simulink model "PFC"  (R2018b)
settings: Solver=VariableStepAuto  StartTime=0.0  StopTime=8  MaxStep=1e-4  RelTol=1e-3
values from neighbouring files (symbols this model uses):
  C = 470e-6    (= 0.00047)    [Parameter_DAD.m]    (also in Parameter_PFC.m = 7.2e-10)
  f_ac = 50    [Parameter_PFC.m]
  I_u = 10    [Parameter_DAD.m]    (also in Parameter_PFC.m)
  L = 50*1e-4    (= 0.005)    [Parameter_DAD.m]    (also in Parameter_PFC.m = 0.003)
  P_u = 5    [Parameter_DAD.m]    (also in Parameter_PFC.m = 0.1)
  R_l = Vdc_trgt^2 / P/eita    (= 400)    [Parameter_PFC.m]
  Vac = 220    [Parameter_PFC.m]
  Vdc_trgt = 400    [Parameter_PFC.m]
libraries: powerlib x16, simulink_extras x2, simulink x1
settings Model: Creator=lenovo  LastModifiedBy=lenovo
settings SFSimCC: SimUseLocalCustomCode=off
settings RTWCC: RTWUseLocalCustomCode=off
settings CodeAppCC: StateflowObjectComments=on

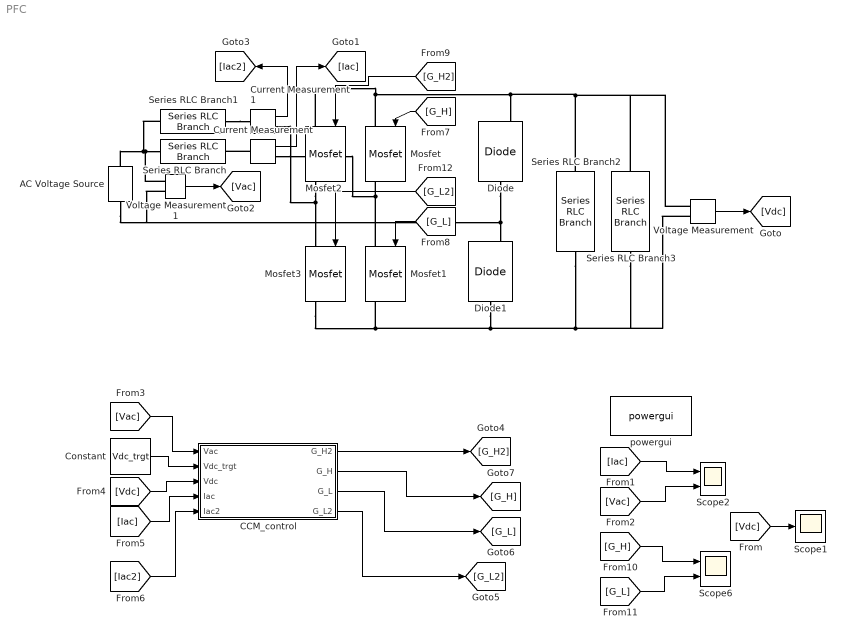
== system PFC ==
  AC Voltage Source : powerlib/Electrical Sources/AC Voltage Source  Amplitude=Vac*sqrt(2)  Phase=0  Frequency=f_ac  SampleTime=0  Measurements=None  BusType=swing  Pref=10e3  Qref=0  Qmin=-inf  Qmax=+inf
      settings: SourceProductName=Simscape Electrical
  CCM_control : Subsystem
  Constant : Constant  Value=Vdc_trgt
  Current Measurement : powerlib/Measurements/Current Measurement  PhasorSimulation=off  OutputType=Complex  PSBequivalent=0
  Current Measurement1 : powerlib/Measurements/Current Measurement  PhasorSimulation=off  OutputType=Complex  PSBequivalent=0
  Diode : powerlib/Power Electronics/Diode  Ron=0.001  Lon=0  Vf=0.8  IC=0  UseSnubber=0  Rs=500  Cs=250e-9  Measurements=on
      settings: SourceProductName=Simscape Electrical
  Diode1 : powerlib/Power Electronics/Diode  Ron=0.001  Lon=0  Vf=0.8  IC=0  UseSnubber=0  Rs=500  Cs=250e-9  Measurements=on
      settings: SourceProductName=Simscape Electrical
  Mosfet{,1..3} (4 alike) : powerlib/Power Electronics/Mosfet  Ron=0.1  Lon=0  Rd=0.01  Vfd=0  IC=0  Rs=1e5  Cs=inf  Measurements=on
      settings: SourceProductName=Simscape Electrical
  Scope1 : Scope
  Scope2 : Scope  NumInputPorts=2
  Scope6 : Scope  NumInputPorts=2
  Series RLC Branch : powerlib/Elements/Series RLC Branch  LConnTagsString=__new0  RConnTagsString=__new0  BranchType=L  Resistance=1  Inductance=L  SetiL0=off  InitialCurrent=0  Capacitance=1e-6  Setx0=off  InitialVoltage=0  Measurements=None
      settings: SourceProductName=Simscape Electrical
  Series RLC Branch1 : powerlib/Elements/Series RLC Branch  LConnTagsString=__new0  RConnTagsString=__new0  BranchType=L  Resistance=1  Inductance=L  SetiL0=off  InitialCurrent=0  Capacitance=1e-6  Setx0=off  InitialVoltage=0  Measurements=None
      settings: SourceProductName=Simscape Electrical
  Series RLC Branch2 : powerlib/Elements/Series RLC Branch  LConnTagsString=__new0  RConnTagsString=__new0  BranchType=C  Resistance=1  Inductance=1e-3  SetiL0=off  InitialCurrent=0  Capacitance=C  Setx0=on  InitialVoltage=0  Measurements=None
      settings: SourceProductName=Simscape Electrical
  Series RLC Branch3 : powerlib/Elements/Series RLC Branch  LConnTagsString=__new0  RConnTagsString=__new0  BranchType=R  Resistance=R_l  Inductance=1e-3  SetiL0=off  InitialCurrent=0  Capacitance=C  Setx0=off  InitialVoltage=0  Measurements=None
      settings: SourceProductName=Simscape Electrical
  Voltage Measurement : powerlib/Measurements/Voltage Measurement  PhasorSimulation=off  OutputType=Complex  PSBequivalent=0
  Voltage Measurement1 : powerlib/Measurements/Voltage Measurement  PhasorSimulation=off  OutputType=Complex  PSBequivalent=0
  powergui : powerlib/powergui  Priority=1  SimulationMode=Discrete  SampleTime=1e-7  frequency=60  Iterations=50  frequencyindice=50  Pbase=100e6  ErrMax=1e-4  UnitsV=kV  UnitsW=MW  buscounter=0  FunctionMessages=off  echomessages=off  EnableUseOfTLC=off  CurrentSourceSwitches=off  DisableSnubberDevices=off  DisableRonSwitches=off  DisableVfSwitches=off  DisplayEquations=off  SolverType=Tustin/Backward Euler (TBE)  Interpol=off  ExternalGateDelay=off  methode=off  Ts=100  x0status=blocks  SPID=off  SwTol=0  HookPort=off  RestoreLinks=warning  ResistiveCurrentMeasurement=off  Frange=[0:2:500]  Ylog=off  Xlog=on  ShowGrid=off  save=off  variable=ZData  structure=0  ZoomFFT=off  StartTime=0.0  cycles=1  DisplayStyle=1  fundamental=60  FreqAxis=off  MaxFrequency=1000  frequencyindicesteady=1  RmsSteady=1  display=off
  wires:
  Voltage Measurement/1 -> [Vdc]
  [Vdc] -> Scope1/1
  Current Measurement/1 -> [Iac]
  [Iac] -> Scope2/1
  Voltage Measurement1/1 -> [Vac]
  [Vac] -> Scope2/2
  [G_H] -> Mosfet/1
  [G_L] -> Mosfet1/1
  [G_H] -> Scope6/1
  [G_L] -> Scope6/2
  [Vac] -> CCM_control/1(Vac)
  Constant/1 -> CCM_control/2(Vdc_trgt)
  [Vdc] -> CCM_control/3(Vdc)
  [Iac] -> CCM_control/4(Iac)
  CCM_control/2(G_H) -> [G_H]
  CCM_control/3(G_L) -> [G_L]
  Current Measurement1/1 -> [Iac2]
  [G_H2] -> Mosfet2/1
  [G_L2] -> Mosfet3/1
  [Iac2] -> CCM_control/5(Iac2)
  CCM_control/1(G_H2) -> [G_H2]
  CCM_control/4(G_L2) -> [G_L2]
  connections:
  Mosfet1/LConn1 -- Current Measurement/RConn1 -- Mosfet/RConn1
  Diode/LConn1 -- Voltage Measurement1/LConn2 -- AC Voltage Source/LConn1 -- Diode1/RConn1
  Diode1/LConn1 -- Voltage Measurement/LConn2 -- Series RLC Branch3/RConn1 -- Series RLC Branch2/RConn1 -- Mosfet3/RConn1 -- Mosfet1/RConn1
  Mosfet/LConn1 -- Mosfet2/LConn1 -- Voltage Measurement/LConn1 -- Series RLC Branch3/LConn1 -- Series RLC Branch2/LConn1 -- Diode/RConn1
  AC Voltage Source/RConn1 -- Series RLC Branch1/LConn1 -- Series RLC Branch/LConn1 -- Voltage Measurement1/LConn1
  Current Measurement/LConn1 -- Series RLC Branch/RConn1
  Series RLC Branch1/RConn1 -- Current Measurement1/LConn1
  Mosfet2/RConn1 -- Mosfet3/LConn1 -- Current Measurement1/RConn1

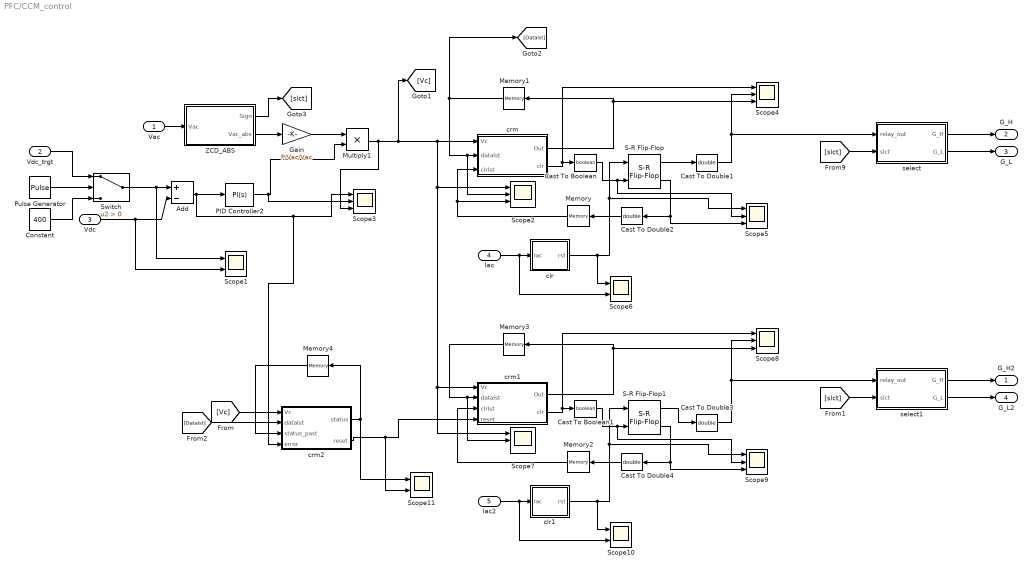
== system PFC/CCM_control ==
  Vac : Inport
  Vdc_trgt : Inport  Port=2
  Vdc : Inport  Port=3
  Iac : Inport  Port=4
  Iac2 : Inport  Port=5
  Add : Sum  Inputs=+-
  Cast To Boolean : DataTypeConversion  OutDataTypeStr=boolean
  Cast To Boolean1 : DataTypeConversion  OutDataTypeStr=boolean
  Cast To Double{1..4} (4 alike) : DataTypeConversion  OutDataTypeStr=double
  Constant : Constant  Value=400
  Gain : Gain  Gain=P/Vac/Vac
  Memory{,1..4} (5 alike) : Memory
  Multiply1 : Product
  PID Controller2 : simulink/Continuous/PID Controller  Controller=PI  Form=Parallel  TimeDomain=Continuous-time  SampleTime=-1  IntegratorMethod=Forward Euler  FilterMethod=Forward Euler  ControllerParametersSource=internal  P=P_u  I=I_u  D=0  UseFilter=on  N=100  TunerSelectOption=Transfer Function Based (PID Tuner App)  InitialConditionSource=internal  InitialConditionForIntegrator=0  InitialConditionForFilter=0  DifferentiatorICPrevScaledInput=0  ExternalReset=none  TrackingMode=off  Kt=1  LimitOutput=on  UpperSaturationLimit=50  LowerSaturationLimit=-10  LinearizeAsGain=off  AntiWindupMode=none  Kb=1  POutMin=[]  POutMax=[]  IOutMin=[]  IOutMax=[]  DOutMin=[]  DOutMax=[]  NOutMin=[]  NOutMax=[]  SumOutMin=[]  SumOutMax=[]  SaturationOutMin=[]  SaturationOutMax=[]  PParamMin=[]  PParamMax=[]  IParamMin=[]  IParamMax=[]  DParamMin=[]  DParamMax=[]  NParamMin=[]  NParamMax=[]  KbParamMin=[]  KbParamMax=[]  KtParamMin=[]  KtParamMax=[]  KbOutMin=[]  KbOutMax=[]  KtOutMin=[]  KtOutMax=[]  IntegratorOutMin=[]  IntegratorOutMax=[]  FilterOutMin=[]  FilterOutMax=[]  SumI1OutMin=[]  SumI1OutMax=[]  SumI2OutMin=[]  SumI2OutMax=[]  SumI3OutMin=[]  SumI3OutMax=[]  SumI4OutMin=[]  SumI4OutMax=[]  SumDOutMin=[]  SumDOutMax=[]  DifferentiatorOutMin=[]  DifferentiatorOutMax=[]  FilterDiffOutCoefMin=[]  FilterDiffOutCoefMax=[]  ReciprocalOutMin=[]  ReciprocalOutMax=[]  SumDenOutMin=[]  SumDenOutMax=[]  SumNumOutMin=[]  SumNumOutMax=[]  DivideOutMin=[]  DivideOutMax=[]  IntegratorContinuousStateAttributes=''  IntegratorStateMustResolveToSignalObject=off  IntegratorRTWStateStorageClass=Auto  FilterContinuousStateAttributes=''  FilterStateMustResolveToSignalObject=off  FilterRTWStateStorageClass=Auto  ParallelPVariant=InternalParameters  IdealPVariant=Disabled  IVariant=InternalParameters  DVariant=Disabled  IntegratorVariant=Continuous  SatVariant=Enabled  AWVariant=Passthrough  PCopyVariant=Disabled  TRVariant=Disabled  FdbkBlocksVariant=Forward  IdealPFdbkVariant=Disabled  SatFdbkVariant=Disabled  DerivativeFilterVariant=Disabled  NVariant=Disabled  NCopyVariant=Disabled_SignalSpec  FilterICVariant=Disabled  IntegratorICVariant=InternalICs  ExternalResetVariant=Disabled  TRSumVariant=Passthrough  SumFdbkVariant=Disabled  SumVariant=Sum_PI
  Pulse Generator : DiscretePulseGenerator  PulseType=Time based  Period=4  PulseWidth=50
  S-R Flip-Flop : simulink_extras/Flip Flops/S-R Flip-Flop  initial_condition=0
  S-R Flip-Flop1 : simulink_extras/Flip Flops/S-R Flip-Flop  initial_condition=0
  Scope{1,6,10..11} (4 alike) : Scope  NumInputPorts=2
  Scope{2..5,7..9} (7 alike) : Scope  NumInputPorts=3
  Switch : Switch  Criteria=u2 > Threshold
  ZCD_ABS : MATLAB Function  TreatAsAtomicUnit=on
  clr : MATLAB Function  TreatAsAtomicUnit=on
  clr1 : MATLAB Function  TreatAsAtomicUnit=on
  crm : MATLAB Function  TreatAsAtomicUnit=on
  crm1 : MATLAB Function  TreatAsAtomicUnit=on
  crm2 : MATLAB Function  TreatAsAtomicUnit=on
  select : MATLAB Function  TreatAsAtomicUnit=on
  select1 : MATLAB Function  TreatAsAtomicUnit=on
  G_H2 : Outport
  G_H : Outport  Port=2
  G_L : Outport  Port=3
  G_L2 : Outport  Port=4
  wires:
  select/2(G_L) -> G_L/1
  ZCD_ABS/2(Vac_abs) -> Gain/1
  select/1(G_H) -> G_H/1
  Add/1 -> crm2/4(error), Scope3/1, PID Controller2/1
  PID Controller2/1 -> Scope3/2, Multiply1/2
  ZCD_ABS/1(Sign) -> [slct]
  Gain/1 -> Multiply1/1
  [slct] -> select/2(slct)
  Vac/1 -> ZCD_ABS/1(Vac)
  Vdc/1 -> Scope1/2, Add/2
  Pulse Generator/1 -> Switch/2
  Constant/1 -> Switch/3
  Vdc_trgt/1 -> Switch/1
  Switch/1 -> Scope1/1, Add/1
  crm/1(Out) -> Scope4/3, Memory1/1
  Memory/1 -> crm/3(clrlst), Scope2/3
  Cast To Double1/1 -> select/1(relay_out), Scope4/2
  Cast To Double2/1 -> Memory/1
  crm/2(clr) -> Scope4/1, Cast To Boolean/1
  Iac/1 -> Scope6/2, clr/1(Iac)
  S-R Flip-Flop/1 -> Cast To Double1/1
  S-R Flip-Flop/2 -> Scope5/3, Cast To Double2/1
  clr/1(rst) -> Scope6/1, Scope5/1, S-R Flip-Flop/1
  Cast To Boolean/1 -> Scope5/2, S-R Flip-Flop/2
  S-R Flip-Flop1/2 -> Scope9/3, Cast To Double4/1
  Cast To Boolean1/1 -> Scope9/2, S-R Flip-Flop1/2
  crm1/2(clr) -> Scope8/1, Cast To Boolean1/1
  clr1/1(rst) -> Scope10/1, Scope9/1, S-R Flip-Flop1/1
  Iac2/1 -> Scope10/2, clr1/1(Iac)
  [slct] -> select1/2(slct)
  select1/2(G_L) -> G_L2/1
  Multiply1/1 -> Scope3/3, [Vc], Scope7/1, crm1/1(Vc), Scope2/1, crm/1(Vc)
  Cast To Double4/1 -> Memory2/1
  select1/1(G_H) -> G_H2/1
  Cast To Double3/1 -> select1/1(relay_out), Scope8/2
  S-R Flip-Flop1/1 -> Cast To Double3/1
  Memory3/1 -> Scope7/2, crm1/2(datalst)
  crm1/1(Out) -> Scope8/3, Memory3/1
  Memory2/1 -> crm1/3(clrlst)
  Memory4/1 -> crm2/3(status_past)
  [Vc] -> crm2/1(Vc)
  Memory1/1 -> [Datalst], Scope2/2, crm/2(datalst)
  [Datalst] -> crm2/2(datalst)
  crm2/1(status) -> Memory4/1, Scope11/1
  crm2/2(reset) -> Scope11/2, crm1/4(reset)

== matlab function PFC/CCM_control/select ==
  data: relay_out input; G_H output; G_L output; slct input
function [G_H, G_L] = fcn(relay_out, slct)


if slct>0.5
    G_L = relay_out;
    G_H = 1-relay_out;
elseif slct<=-0.5
    G_L = 1-relay_out;
    G_H = relay_out; 
else
    G_L = 0;
    G_H = 0; 
end    
end

== matlab function PFC/CCM_control/ZCD_ABS ==
  data: Vac input; Sign output; Vac_abs output
function [Sign, Vac_abs] = fcn(Vac)
Vac_abs = abs(Vac);
Sign = sign(Vac);
end

== matlab function PFC/CCM_control/crm ==
  data: Vc input size=1; Out output size=1; datalst input size=1; clr output size=1; clrlst input size=1
function [Out, clr] = fcn(Vc, datalst, clrlst)
if Vc <= datalst
    clr = 1;
else
    clr = 0;
end
%clr = bool(clr);
if clrlst == 1
    Out = 0;
else
    Out = datalst + 0.1;
end

end

== matlab function PFC/CCM_control/clr ==
  data: Iac input; rst output
function rst = fcn(Iac)
temp = abs(Iac);
rst = (temp < 0.1);
end

== matlab function PFC/CCM_control/clr1 ==
  data: Iac input; rst output
function rst = fcn(Iac)
temp = abs(Iac);
rst = (temp < 0.1);
end

== matlab function PFC/CCM_control/crm1 ==
  data: Vc input size=1; Out output size=1; datalst input size=1; clr output size=1; clrlst input size=1; reset input
function [Out, clr] = fcn(Vc, datalst, clrlst, reset)
if reset == 1
    Out = 0;
    clr = 0;
else
    if Vc <= datalst
        clr = 1;
    else
        clr = 0;
    end
    %clr = bool(clr);
    if clrlst == 1
        Out = 0;
    else
        Out = datalst + 0.1;
    end
end
end

== matlab function PFC/CCM_control/select1 ==
  data: relay_out input; G_H output; G_L output; slct input
function [G_H, G_L] = fcn(relay_out, slct)


if slct>0.5
    G_L = relay_out;
    G_H = 1-relay_out;
elseif slct<=-0.5
    G_L = 1-relay_out;
    G_H = relay_out; 
else
    G_L = 0;
    G_H = 0; 
end    
end

== matlab function PFC/CCM_control/crm2 ==
  data: Vc input size=1; status output size=1; datalst input size=1; reset output size=1; status_past input size=1; error input
function [status, reset] = fcn(Vc, datalst, status_past, error)
Error = abs(error);
if (datalst < 0.7*Vc|| Error > 10) && status_past==0
    status = 0;
else
    status = 1;
end
reset = 1-status;
end
